simulink model "test_car_2021b"  (R2021b)
settings: Solver=ode15s  StartTime=0.0  StopTime=10  RelTol=1e-3
model workspace (MAT data in the model file):
  Ah = 5200
  B = 0.00011
  J = 4.7e-05
  K = 0.01
  L = 0.01
  Ld = 0.007
  Lq = 0.007
  Mspwm = 0.9
  R = 0.01
  Ra = 2.98
  af = 0.57
  b = 0.1
  c1 = 0.001947
  cdrag = 0.37
  k0 = 380
  k2 = 2
  k3 = 20
  k4 = -5
  mass = 300
  p = 2
  pm = 0.125
  rho = 1.18
  socInit = 1
  vnom = 400
  wheelRadius = 0.3
settings Model: Creator=sansh  LastModifiedBy=jw3019
settings SolverCC: AlgebraicLoopSolver=TrustRegion
settings DataIOCC: ReturnWorkspaceOutputs=off
settings DebuggingCC: SFMachineParentedDataDiag=warning  ArithmeticOperatorsInVariantConditions=warning
settings SFSimCC: SimUseLocalCustomCode=off  CustomCodeUndefinedFunction=UseInterfaceOnly
settings RTWCC: RTWUseLocalCustomCode=off  DLArmComputeVersion=20.02.1
settings CodeAppCC: StateflowObjectComments=on

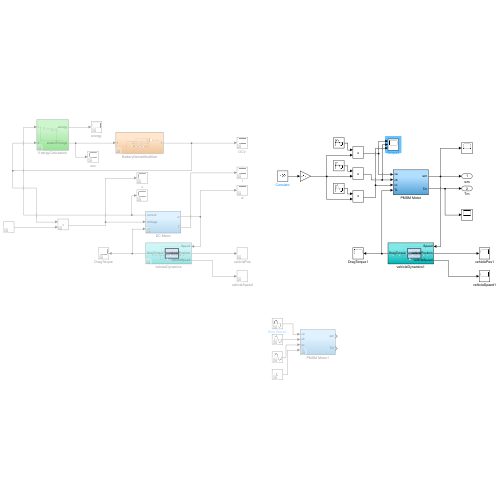
[thumbnail: Simulink's stored preview of the top-level diagram]
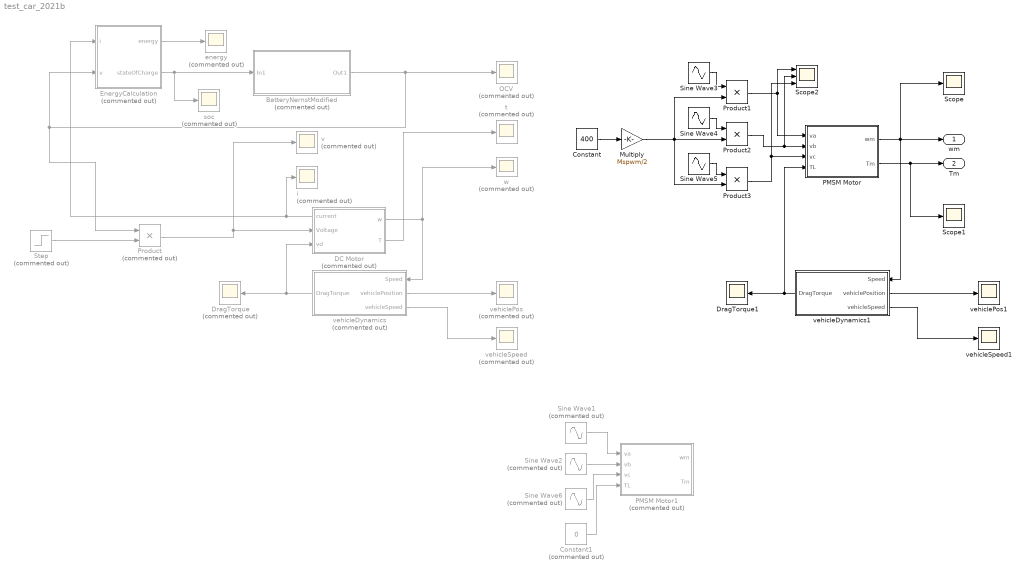
== system test_car_2021b ==
  BatteryNernstModified : Subsystem  Commented=on
  Constant : Constant  Value=400
  Constant1 : Constant  Commented=on  Value=0
  DC Motor : Subsystem  Commented=on
      settings: PortSchema="{\"entries\":[{\"content\":{\"sides\":[{\"content\":{\"connectorIds\":[\"Out3\",\"In1\",\"In2\"]},\"type\":\"ConnectorPlacement.EquallySpacedRectSide\",\"uuid\":\"b276cc4c-6e56-4956-8f44-003124433d7e\"},{\"content\":{\"connectorIds\":[\"Out1\",\"Out2\"],\"side\":\"RIGHT\"},\"type\":\"ConnectorPlacement.EquallySpacedRectSide\",\"uuid\":\"98d555dc-4bec-4179-83d1-7f47ef529afe\"},{\"content\":{\"connectorIds\":[],\"side\":\"TOP\"},\"type\":\"ConnectorPlacement.EquallySpacedRectSide\",\"uuid\":\"179053d8-aed3-445b-8bde-cf864afeeb53\"}]},\"type\":\"ConnectorPlacement.EquallySpacedConnector\",\"uuid\":\"b402df6a-fe5a-46c9-a6de-67aaf8332b13\"}],\"packageUris\":[\"http://schema.mathworks.com/mf0/Connector/R2020b\"],\"version\":\"1.0\"}"
  DragTorque : Scope  Commented=on
  DragTorque1 : Scope
  EnergyCalculation : Subsystem  Commented=on
  Multiply : Gain  Gain=Mspwm/2
  OCV : Scope  Commented=on
  PMSM Motor : Subsystem
  PMSM Motor1 : Subsystem  Commented=on
  Product : Product  Commented=on
  Product1 : Product
  Product2 : Product
  Product3 : Product
  Scope : Scope
  Scope1 : Scope
  Scope2 : Scope  NumInputPorts=3
  Sine Wave1 : Sin  Commented=on  Amplitude=240  Frequency=2*pi*50  SampleTime=0.001  VectorParams1D=off
  Sine Wave2 : Sin  Commented=on  Amplitude=240  Frequency=2*pi*50  Phase=-(2*pi)/3  SampleTime=0.001  VectorParams1D=off
  Sine Wave3 : Sin  Frequency=2*pi*50  SampleTime=0.001  VectorParams1D=off
  Sine Wave4 : Sin  Frequency=2*pi*50  Phase=-(2*pi)/3  SampleTime=0.001
  Sine Wave5 : Sin  Frequency=2*pi*50  Phase=(2*pi)/3  SampleTime=0.001
  Sine Wave6 : Sin  Commented=on  Amplitude=240  Frequency=2*pi*50  Phase=(2*pi)/3  SampleTime=0.001  VectorParams1D=off
  Step : Step  Commented=on  SampleTime=0
  energy : Scope  Commented=on
  i : Scope  Commented=on
  soc : Scope  Commented=on
  t : Scope  Commented=on
  v : Scope  Commented=on
  vehicleDynamics : Subsystem  Commented=on
      settings: PortSchema="{\"entries\":[{\"content\":{\"sides\":[{\"content\":{\"connectorIds\":[\"In1\",\"Out2\",\"Out3\"]},\"type\":\"ConnectorPlacement.EquallySpacedRectSide\",\"uuid\":\"07ecf1cb-0d5c-4608-88cc-e61117b79db0\"},{\"content\":{\"connectorIds\":[\"Out1\"],\"side\":\"RIGHT\"},\"type\":\"ConnectorPlacement.EquallySpacedRectSide\",\"uuid\":\"003f7a32-9b2b-44d7-acb6-981f8f38bf0d\"},{\"content\":{\"connectorIds\":[],\"side\":\"TOP\"},\"type\":\"ConnectorPlacement.EquallySpacedRectSide\",\"uuid\":\"864d97b5-3a75-4ab5-b9c0-20b3f38956ab\"}]},\"type\":\"ConnectorPlacement.EquallySpacedConnector\",\"uuid\":\"7c02dec8-5acc-4a8e-8ac6-d1d16052955e\"}],\"packageUris\":[\"http://schema.mathworks.com/mf0/Connector/R2020b\"],\"version\":\"1.0\"}"
  vehicleDynamics1 : Subsystem
      settings: PortSchema="{\"entries\":[{\"content\":{\"sides\":[{\"content\":{\"connectorIds\":[\"In1\",\"Out2\",\"Out3\"]},\"type\":\"ConnectorPlacement.EquallySpacedRectSide\",\"uuid\":\"07ecf1cb-0d5c-4608-88cc-e61117b79db0\"},{\"content\":{\"connectorIds\":[\"Out1\"],\"side\":\"RIGHT\"},\"type\":\"ConnectorPlacement.EquallySpacedRectSide\",\"uuid\":\"003f7a32-9b2b-44d7-acb6-981f8f38bf0d\"},{\"content\":{\"connectorIds\":[],\"side\":\"TOP\"},\"type\":\"ConnectorPlacement.EquallySpacedRectSide\",\"uuid\":\"864d97b5-3a75-4ab5-b9c0-20b3f38956ab\"}]},\"type\":\"ConnectorPlacement.EquallySpacedConnector\",\"uuid\":\"7c02dec8-5acc-4a8e-8ac6-d1d16052955e\"}],\"packageUris\":[\"http://schema.mathworks.com/mf0/Connector/R2020b\"],\"version\":\"1.0\"}"
  vehiclePos : Scope  Commented=on
  vehiclePos1 : Scope
  vehicleSpeed : Scope  Commented=on
  vehicleSpeed1 : Scope
  w : Scope  Commented=on
  wm : Outport
  Tm : Outport  Port=2
  wires:
  DC Motor/1(w) -> vehicleDynamics/1(Speed), w/1
  DC Motor/3(current) -> EnergyCalculation/1(i), i/1
  DC Motor/2(T) -> t/1
  vehicleDynamics/1(DragTorque) -> DC Motor/2(vd), DragTorque/1
  vehicleDynamics/2(vehiclePosition) -> vehiclePos/1
  vehicleDynamics/3(vehicleSpeed) -> vehicleSpeed/1
  EnergyCalculation/1(energy) -> energy/1
  EnergyCalculation/2(stateOfCharge) -> BatteryNernstModified/1(In1), soc/1
  Step/1 -> Product/2
  Product/1 -> v/1, DC Motor/1(Voltage)
  BatteryNernstModified/1(Out1) -> OCV/1, EnergyCalculation/2(v), Product/1
  PMSM Motor/1(wm) -> wm/1, Scope/1, vehicleDynamics1/1(Speed)
  PMSM Motor/2(Tm) -> Scope1/1, Tm/1
  Multiply/1 -> Product3/2, Product2/2, Product1/2
  Sine Wave3/1 -> Product1/1
  Sine Wave4/1 -> Product2/1
  Sine Wave5/1 -> Product3/1
  Product1/1 -> PMSM Motor/1(va), Scope2/1
  Product2/1 -> Scope2/2, PMSM Motor/2(vb)
  Product3/1 -> Scope2/3, PMSM Motor/3(vc)
  Constant/1 -> Multiply/1
  vehicleDynamics1/2(vehiclePosition) -> vehiclePos1/1
  vehicleDynamics1/1(DragTorque) -> PMSM Motor/4(TL), DragTorque1/1
  vehicleDynamics1/3(vehicleSpeed) -> vehicleSpeed1/1
  Sine Wave1/1 -> PMSM Motor1/1(va)
  Sine Wave2/1 -> PMSM Motor1/2(vb)
  Sine Wave6/1 -> PMSM Motor1/3(vc)
  Constant1/1 -> PMSM Motor1/4(TL)

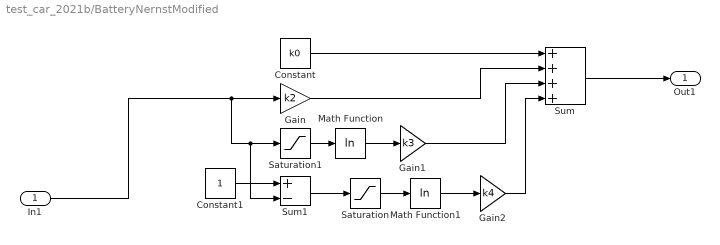
== system test_car_2021b/BatteryNernstModified ==
  In1 : Inport
  Constant : Constant  Value=k0
  Constant1 : Constant
  Gain : Gain  Gain=k2
  Gain1 : Gain  Gain=k3
  Gain2 : Gain  Gain=k4
  Math Function : Math  Operator=log  SaturateOnIntegerOverflow=on
  Math Function1 : Math  Operator=log  SaturateOnIntegerOverflow=on
  Saturation : Saturate  UpperLimit=1  LowerLimit=0.01
  Saturation1 : Saturate  UpperLimit=1  LowerLimit=0.01
  Sum : Sum  Inputs=++++
  Sum1 : Sum  Inputs=+-
  Out1 : Outport
  wires:
  Gain2/1 -> Sum/4
  Sum1/1 -> Saturation/1
  Saturation/1 -> Math Function1/1
  Constant/1 -> Sum/1
  Math Function1/1 -> Gain2/1
  Math Function/1 -> Gain1/1
  Constant1/1 -> Sum1/1
  Gain1/1 -> Sum/3
  Saturation1/1 -> Math Function/1
  Sum/1 -> Out1/1
  Gain/1 -> Sum/2
  In1/1 -> Saturation1/1, Sum1/2, Gain/1

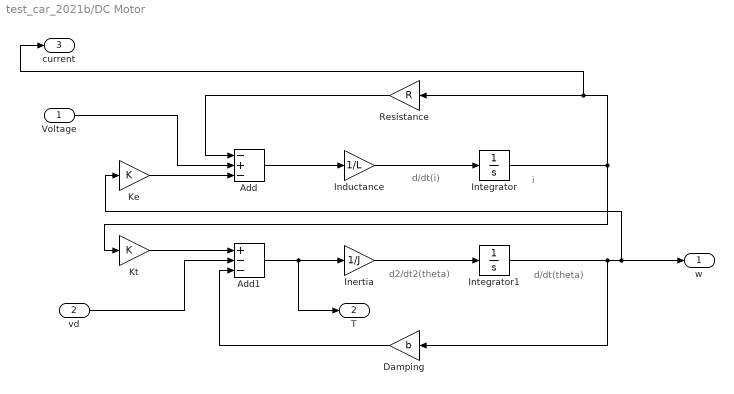
== system test_car_2021b/DC Motor ==
  note: i
  note: d/dt(i)
  note: d/dt(theta)
  note: d2/dt2(theta)
  Voltage : Inport
  vd : Inport  Port=2
  Add : Sum  Inputs=-+-
  Add1 : Sum  Inputs=+--
  Damping : Gain  Gain=b
  Inductance : Gain  Gain=1/L
  Inertia : Gain  Gain=1/J
  Integrator : Integrator
  Integrator1 : Integrator
  Ke : Gain  Gain=K
  Kt : Gain  Gain=K
  Resistance : Gain  Gain=R
  w : Outport
  T : Outport  Port=2
  current : Outport  Port=3
  wires:
  Inductance/1 -> Integrator/1
  Integrator1/1 -> Damping/1, w/1, Ke/1
  Inertia/1 -> Integrator1/1
  Integrator/1 -> current/1, Resistance/1, Kt/1
  Kt/1 -> Add1/1
  Voltage/1 -> Add/2
  Resistance/1 -> Add/1
  Damping/1 -> Add1/3
  Ke/1 -> Add/3
  Add/1 -> Inductance/1
  Add1/1 -> T/1, Inertia/1
  vd/1 -> Add1/2

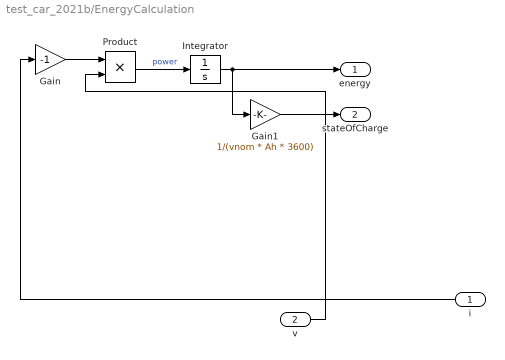
== system test_car_2021b/EnergyCalculation ==
  i : Inport
  v : Inport  Port=2
  Gain : Gain  Gain=-1
  Gain1 : Gain  Gain=1/(vnom * Ah * 3600)
  Integrator : Integrator  InitialCondition=socInit * vnom * Ah * 3600
  Product : Product
  energy : Outport
  stateOfCharge : Outport  Port=2
  wires:
  v/1 -> Product/2
  i/1 -> Gain/1
  Product/1 -> Integrator/1  "power"
  Gain1/1 -> stateOfCharge/1
  Gain/1 -> Product/1
  Integrator/1 -> energy/1, Gain1/1

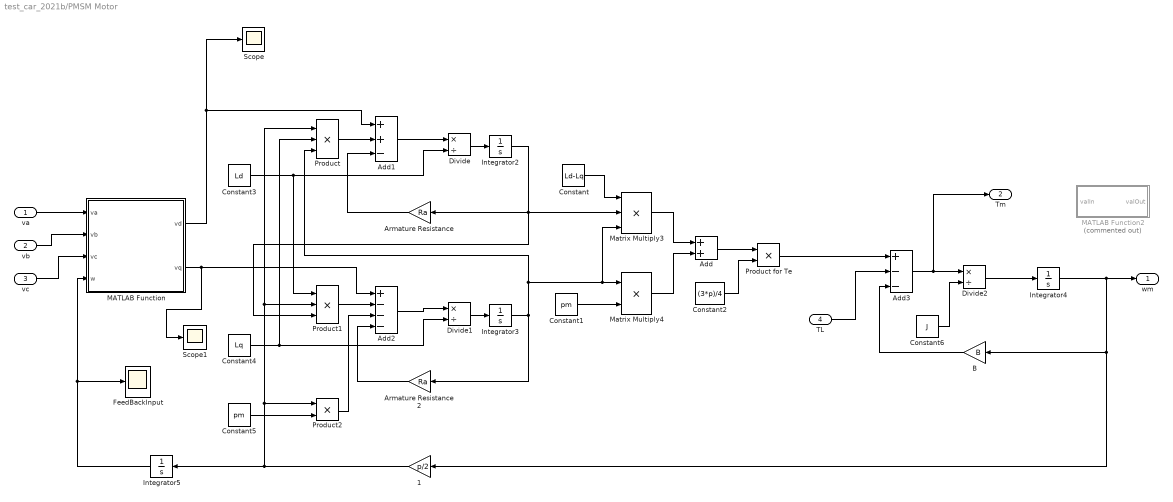
== system test_car_2021b/PMSM Motor ==
  va : Inport
  vb : Inport  Port=2
  vc : Inport  Port=3
  TL : Inport  Port=4
  1 : Gain  Gain=p/2
  Add : Sum
  Add1 : Sum  Inputs=++-
  Add2 : Sum  Inputs=+---
  Add3 : Sum  Inputs=+--
  Armature Resistance : Gain  Gain=Ra
  Armature Resistance 2 : Gain  Gain=Ra
  B : Gain  Gain=B
  Constant : Constant  Value=Ld-Lq
  Constant1 : Constant  Value=pm
  Constant2 : Constant  Value=(3*p)/4
  Constant3 : Constant  Value=Ld
  Constant4 : Constant  Value=Lq
  Constant5 : Constant  Value=pm
  Constant6 : Constant  Value=J
  Divide : Product  Inputs=*/
  Divide1 : Product  Inputs=*/
  Divide2 : Product  Inputs=*/
  FeedBackInput : Scope
  Integrator{2..5} (4 alike) : Integrator
  MATLAB Function : MATLAB Function  TreatAsAtomicUnit=on
  MATLAB Function2 : MATLAB Function  Commented=on  TreatAsAtomicUnit=on
  Matrix Multiply3 : Product  Inputs=3
  Matrix Multiply4 : Product
  Product : Product  Inputs=3
  Product for Te : Product
  Product1 : Product  Inputs=3
  Product2 : Product
  Scope : Scope
  Scope1 : Scope
  wm : Outport
  Tm : Outport  Port=2
  wires:
  Constant/1 -> Matrix Multiply3/1
  Integrator3/1 -> Matrix Multiply3/3, Matrix Multiply4/1, Product/3, Armature Resistance 2/1
  Constant1/1 -> Matrix Multiply4/2
  Matrix Multiply3/1 -> Add/1
  Matrix Multiply4/1 -> Add/2
  Add/1 -> Product for Te/1
  Constant2/1 -> Product for Te/2
  MATLAB Function/1(vd) -> Scope/1, Add1/1
  1/1 -> Integrator5/1, Product/1, Product1/2, Product2/1
  Add1/1 -> Divide/1
  Constant3/1 -> Product1/1, Divide/2
  Divide/1 -> Integrator2/1
  Product/1 -> Add1/2
  Integrator2/1 -> Matrix Multiply3/2, Product1/3, Armature Resistance/1
  Armature Resistance 2/1 -> Add2/4
  MATLAB Function/2(vq) -> Scope1/1, Add2/1
  Divide1/1 -> Integrator3/1
  Add2/1 -> Divide1/1
  Constant4/1 -> Divide1/2, Product/2
  Product1/1 -> Add2/2
  Armature Resistance/1 -> Add1/3
  Constant5/1 -> Product2/2
  Product2/1 -> Add2/3
  Constant6/1 -> Divide2/2
  Add3/1 -> Tm/1, Divide2/1
  B/1 -> Add3/3
  Integrator4/1 -> 1/1, B/1, wm/1
  Product for Te/1 -> Add3/1
  TL/1 -> Add3/2
  Integrator5/1 -> MATLAB Function/4(w), FeedBackInput/1
  va/1 -> MATLAB Function/1(va)
  vb/1 -> MATLAB Function/2(vb)
  vc/1 -> MATLAB Function/3(vc)
  Divide2/1 -> Integrator4/1

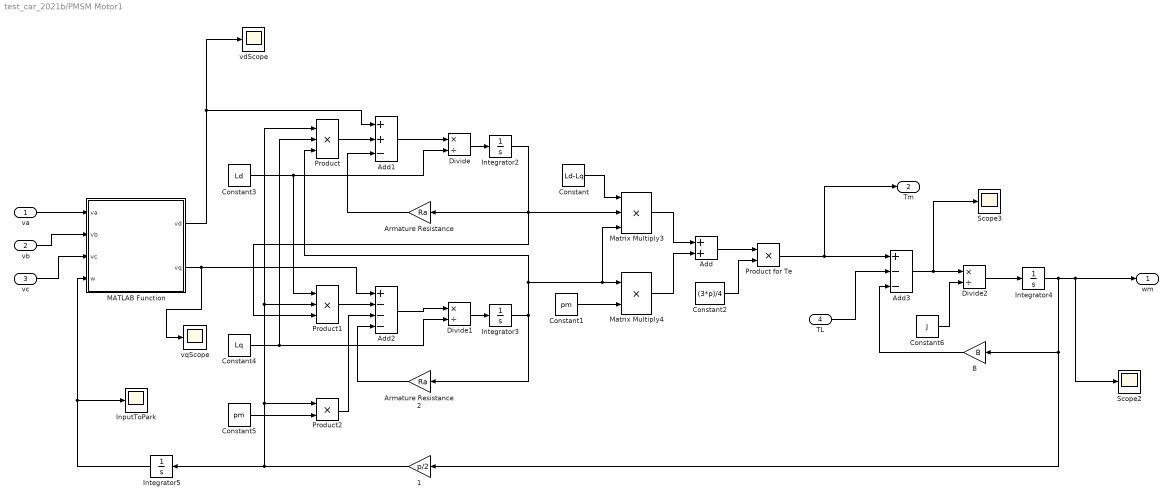
== system test_car_2021b/PMSM Motor1 ==
  va : Inport
  vb : Inport  Port=2
  vc : Inport  Port=3
  TL : Inport  Port=4
  1 : Gain  Gain=p/2
  Add : Sum
  Add1 : Sum  Inputs=++-
  Add2 : Sum  Inputs=+---
  Add3 : Sum  Inputs=+--
  Armature Resistance : Gain  Gain=Ra
  Armature Resistance 2 : Gain  Gain=Ra
  B : Gain  Gain=B
  Constant : Constant  Value=Ld-Lq
  Constant1 : Constant  Value=pm
  Constant2 : Constant  Value=(3*p)/4
  Constant3 : Constant  Value=Ld
  Constant4 : Constant  Value=Lq
  Constant5 : Constant  Value=pm
  Constant6 : Constant  Value=J
  Divide : Product  Inputs=*/
  Divide1 : Product  Inputs=*/
  Divide2 : Product  Inputs=*/
  InputToPark : Scope
  Integrator{2..5} (4 alike) : Integrator
  MATLAB Function : MATLAB Function  TreatAsAtomicUnit=on
  Matrix Multiply3 : Product  Inputs=3
  Matrix Multiply4 : Product
  Product : Product  Inputs=3
  Product for Te : Product
  Product1 : Product  Inputs=3
  Product2 : Product
  Scope2 : Scope
  Scope3 : Scope
  vdScope : Scope
  vqScope : Scope
  wm : Outport
  Tm : Outport  Port=2
  wires:
  Constant/1 -> Matrix Multiply3/1
  Integrator3/1 -> Matrix Multiply3/3, Matrix Multiply4/1, Product/3, Armature Resistance 2/1
  Constant1/1 -> Matrix Multiply4/2
  Matrix Multiply3/1 -> Add/1
  Matrix Multiply4/1 -> Add/2
  Add/1 -> Product for Te/1
  Constant2/1 -> Product for Te/2
  MATLAB Function/1(vd) -> vdScope/1, Add1/1
  1/1 -> Integrator5/1, Product/1, Product1/2, Product2/1
  Add1/1 -> Divide/1
  Constant3/1 -> Product1/1, Divide/2
  Divide/1 -> Integrator2/1
  Product/1 -> Add1/2
  Integrator2/1 -> Matrix Multiply3/2, Product1/3, Armature Resistance/1
  Armature Resistance 2/1 -> Add2/4
  MATLAB Function/2(vq) -> vqScope/1, Add2/1
  Divide1/1 -> Integrator3/1
  Add2/1 -> Divide1/1
  Constant4/1 -> Divide1/2, Product/2
  Product1/1 -> Add2/2
  Armature Resistance/1 -> Add1/3
  Constant5/1 -> Product2/2
  Product2/1 -> Add2/3
  Divide2/1 -> Integrator4/1
  Constant6/1 -> Divide2/2
  Add3/1 -> Scope3/1, Divide2/1
  B/1 -> Add3/3
  Integrator4/1 -> 1/1, B/1, Scope2/1, wm/1
  Product for Te/1 -> Tm/1, Add3/1
  TL/1 -> Add3/2
  Integrator5/1 -> InputToPark/1, MATLAB Function/4(w)
  va/1 -> MATLAB Function/1(va)
  vb/1 -> MATLAB Function/2(vb)
  vc/1 -> MATLAB Function/3(vc)

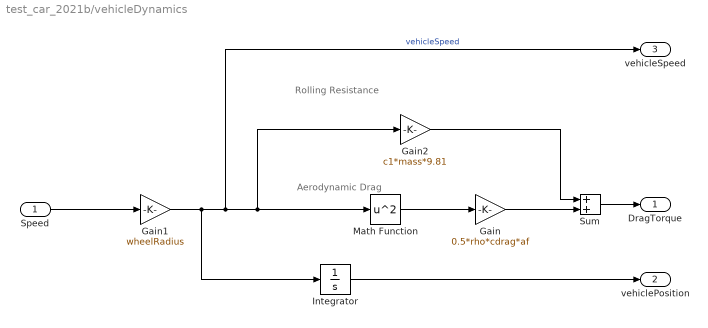
== system test_car_2021b/vehicleDynamics ==
  note: Rolling Resistance
  note: Aerodynamic Drag
  Speed : Inport
  Gain : Gain  Gain=0.5*rho*cdrag*af
  Gain1 : Gain  Gain=wheelRadius
  Gain2 : Gain  Gain=c1*mass*9.81
  Integrator : Integrator
  Math Function : Math  Operator=square  SaturateOnIntegerOverflow=on
  Sum : Sum
  DragTorque : Outport
  vehiclePosition : Outport  Port=2
  vehicleSpeed : Outport  Port=3
  wires:
  Gain/1 -> Sum/2
  Speed/1 -> Gain1/1
  Math Function/1 -> Gain/1
  Gain1/1 -> Gain2/1, Math Function/1, vehicleSpeed/1, Integrator/1  "vehicleSpeed"
  Integrator/1 -> vehiclePosition/1
  Sum/1 -> DragTorque/1
  Gain2/1 -> Sum/1

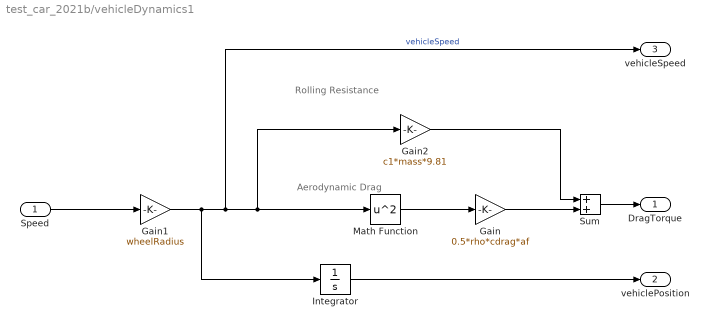
== system test_car_2021b/vehicleDynamics1 ==
  note: Rolling Resistance
  note: Aerodynamic Drag
  Speed : Inport
  Gain : Gain  Gain=0.5*rho*cdrag*af
  Gain1 : Gain  Gain=wheelRadius
  Gain2 : Gain  Gain=c1*mass*9.81
  Integrator : Integrator
  Math Function : Math  Operator=square  SaturateOnIntegerOverflow=on
  Sum : Sum
  DragTorque : Outport
  vehiclePosition : Outport  Port=2
  vehicleSpeed : Outport  Port=3
  wires:
  Gain/1 -> Sum/2
  Speed/1 -> Gain1/1
  Math Function/1 -> Gain/1
  Gain1/1 -> Gain2/1, Math Function/1, vehicleSpeed/1, Integrator/1  "vehicleSpeed"
  Integrator/1 -> vehiclePosition/1
  Sum/1 -> DragTorque/1
  Gain2/1 -> Sum/1

== matlab function test_car_2021b/PMSM Motor1/MATLAB Function ==
  data: va input; vd output; vb input; vc input; vq output; w input
function [vd, vq]= PCTransform(va, vb, vc, w)
vd = (2*(va*sin(w) + vb*sin(w - 2*pi/3) + vc*sin(w + 2*pi/3)))/3;
vq = (2*(va*cos(w) + vb*cos(w - 2*pi/3) + vc*cos(w + 2*pi/3)))/3;

== matlab function test_car_2021b/PMSM Motor/MATLAB Function ==
  data: va input; vd output; vb input; vc input; vq output; w input
function [vd, vq]= PCTransform(va, vb, vc, w)
vd = (2*(va*sin(w) + vb*sin(w - 2*pi/3) + vc*sin(w + 2*pi/3)))/3;
vq = (2*(va*cos(w) + vb*cos(w - 2*pi/3) + vc*cos(w + 2*pi/3)))/3;

== matlab function test_car_2021b/PMSM Motor/MATLAB Function2 ==
  data: valIn input; valOut output
function valOut = ValCheck(valIn)
valIn
if valIn == 0
    valOut = 0.001;
elseif valIn ~= 0
    valOut = valIn;
end
